simulink model "unicycle"  (R2025b)
settings: Solver=VariableStepAuto  StartTime=0.0  StopTime=10.0  RelTol=1e-3
values from neighbouring files (symbols this model uses):
  L = 0.3    [unicycle_init.m]
undefined symbols (not defined in the file or in its folder): R
settings Model: Creator=cardaver  LastModifiedBy=cardaver

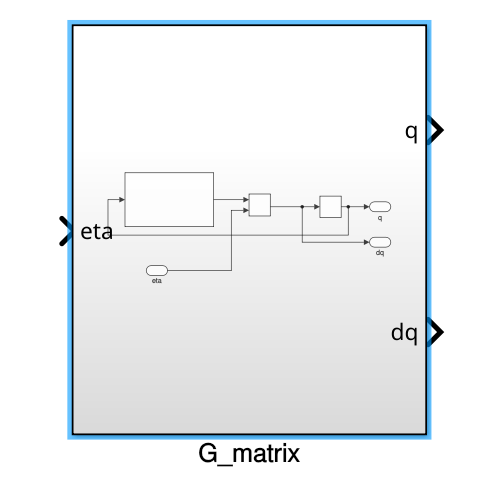
[thumbnail: Simulink's stored preview of the top-level diagram]
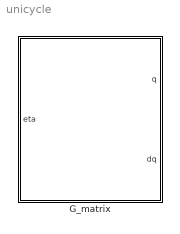
== system unicycle ==
  G_matrix : Subsystem

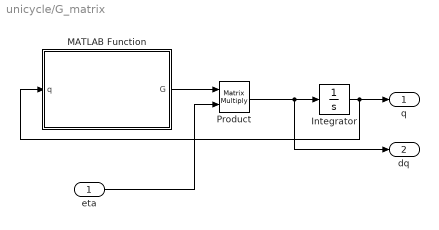
== system unicycle/G_matrix ==
  eta : Inport  PortDimensions=2
  Integrator : Integrator
  MATLAB Function : MATLAB Function  TreatAsAtomicUnit=on
  Product : Product  Multiplication=Matrix(*)
  q : Outport  PortDimensions=5
  dq : Outport  Port=2  PortDimensions=5
  wires:
  eta/1 -> Product/2
  Integrator/1 -> q/1, MATLAB Function/1(q)
  MATLAB Function/1(G) -> Product/1
  Product/1 -> dq/1, Integrator/1

== matlab function unicycle/G_matrix/MATLAB Function ==
  data: q input; G output; L parameter; R parameter
function G = fcn(q, L, R)

theta = q(3);

G = [cos(theta), cos(theta); 
    sin(theta), sin(theta); 
    1/L, -1/L; 
    2/R, 0; 
    0, 2/R];
